simulink model "srinu_ver6"  (R2020b)
settings: Solver=ode15s  StartTime=0.0  StopTime=50  MaxStep=1.0  RelTol=1e-3
undefined symbols (not defined in the file): fn_1, jw_1, m_1, mu_1, r_1, slip_1, v_1, w
libraries: pid_lib x1
settings Model: Creator=K E S SRINIVAS  LastModifiedBy=K E S SRINIVAS

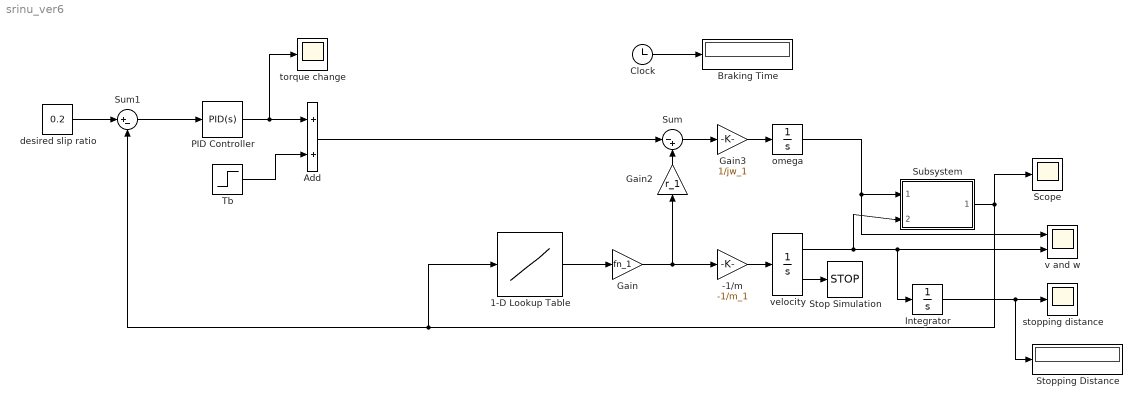
== system srinu_ver6 ==
  -1/m : Gain  Gain=-1/m_1
  1-D Lookup Table : Lookup_n-D  NumberOfTableDimensions=1  BreakpointsForDimension1=slip_1  Table=mu_1  InternalRulePriority=Speed  RndMeth=Simplest  InputSameDT=on
  Add : Sum
  Braking Time : Display
  Clock : Clock
  Gain : Gain  Gain=fn_1
  Gain2 : Gain  Gain=r_1
  Gain3 : Gain  Gain=1/jw_1
  Integrator : Integrator
  PID Controller : pid_lib/PID Controller  Controller=PID  Form=Parallel  TimeDomain=Continuous-time  UseExternalTs=off  SampleTime=-1  IntegratorMethod=Forward Euler  FilterMethod=Forward Euler  ControllerParametersSource=internal  P=250  I=10  D=5  UseFilter=on  N=100  TunerSelectOption=Transfer Function Based (PID Tuner App)  InitialConditionSource=internal  InitialConditionForIntegrator=0  InitialConditionForFilter=0  DifferentiatorICPrevScaledInput=0  ExternalReset=none  TrackingMode=off  Kt=1  LimitOutput=off  SatLimitsSource=internal  UpperSaturationLimit=inf  LowerSaturationLimit=-inf  LinearizeAsGain=on  AntiWindupMode=none  Kb=1  POutMin=[]  POutMax=[]  IOutMin=[]  IOutMax=[]  DOutMin=[]  DOutMax=[]  NOutMin=[]  NOutMax=[]  SumOutMin=[]  SumOutMax=[]  SaturationOutMin=[]  SaturationOutMax=[]  PParamMin=[]  PParamMax=[]  IParamMin=[]  IParamMax=[]  DParamMin=[]  DParamMax=[]  NParamMin=[]  NParamMax=[]  KbParamMin=[]  KbParamMax=[]  KtParamMin=[]  KtParamMax=[]  KbOutMin=[]  KbOutMax=[]  KtOutMin=[]  KtOutMax=[]  IntegratorOutMin=[]  IntegratorOutMax=[]  FilterOutMin=[]  FilterOutMax=[]  SumI1OutMin=[]  SumI1OutMax=[]  SumI2OutMin=[]  SumI2OutMax=[]  SumI3OutMin=[]  SumI3OutMax=[]  SumI4OutMin=[]  SumI4OutMax=[]  SumDOutMin=[]  SumDOutMax=[]  DifferentiatorOutMin=[]  DifferentiatorOutMax=[]  FilterDiffOutCoefMin=[]  FilterDiffOutCoefMax=[]  ReciprocalOutMin=[]  ReciprocalOutMax=[]  SumDenOutMin=[]  SumDenOutMax=[]  SumNumOutMin=[]  SumNumOutMax=[]  DivideOutMin=[]  DivideOutMax=[]  UdiffTsProdOutMin=[]  UdiffTsProdOutMax=[]  NTsProdOutMin=[]  NTsProdOutMax=[]  UintegralTsProdOutMin=[]  UintegralTsProdOutMax=[]  UngainTsProdOutMin=[]  UngainTsProdOutMax=[]  IntegratorContinuousStateAttributes=''  IntegratorStateMustResolveToSignalObject=off  IntegratorRTWStateStorageClass=Auto  FilterContinuousStateAttributes=''  FilterStateMustResolveToSignalObject=off  FilterRTWStateStorageClass=Auto  ParallelPVariant=InternalParameters  IdealPVariant=Disabled  IVariant=InternalParameters  DVariant=InternalParameters  IntegratorVariant=Continuous  SatVariant=Disabled  AWVariant=Passthrough  PCopyVariant=Disabled  TRVariant=Disabled  FdbkBlocksVariant=Forward  IdealPFdbkVariant=Disabled  SatFdbkVariant=Disabled  DerivativeFilterVariant=ContFilter  NVariant=InternalParameters  NCopyVariant=Disabled  FilterICVariant=InternalICsFilter  IntegratorICVariant=InternalICs  ExternalResetVariant=Disabled  TRSumVariant=Passthrough  SumFdbkVariant=Disabled  SumVariant=Sum_PID  TsampFilterVariant=InternalTs  TsampNgainVariant=Passthrough  TsampIntegralVariant=Passthrough  ExternalSaturationOutDataTypeStr=Inherit: Same as second input
  Scope : Scope
  Stop Simulation : Stop
  Stopping Distance : Display
  Subsystem : Subsystem
  Sum : Sum  Inputs=|-+
  Sum1 : Sum  Inputs=|+-
  Tb : Step  Time=0  After=0  SampleTime=0
  desired slip ratio : Constant  Value=0.2
  omega : Integrator  InitialCondition=w  LimitOutput=on  UpperSaturationLimit=1000  LowerSaturationLimit=0
  stopping distance : Scope
  torque change : Scope
  v and w : Scope  NumInputPorts=2
  velocity : Integrator  InitialCondition=v_1  LimitOutput=on  UpperSaturationLimit=1000  LowerSaturationLimit=0  ShowSaturationPort=on
  wires:
  Gain/1 -> Gain2/1, -1/m/1
  Gain2/1 -> Sum/2
  Add/1 -> Sum/1
  Tb/1 -> Add/2
  PID Controller/1 -> torque change/1, Add/1
  Sum/1 -> Gain3/1
  Gain3/1 -> omega/1
  -1/m/1 -> velocity/1
  velocity/1 -> Integrator/1, v and w/2, Subsystem/2(velocity)
  1-D Lookup Table/1 -> Gain/1
  velocity/2 -> Stop Simulation/1
  Subsystem/1(slip ratio) -> Scope/1, 1-D Lookup Table/1, Sum1/2
  Integrator/1 -> Stopping Distance/1, stopping distance/1
  Clock/1 -> Braking Time/1
  Sum1/1 -> PID Controller/1
  desired slip ratio/1 -> Sum1/1
  omega/1 -> v and w/1, Subsystem/1(omega)

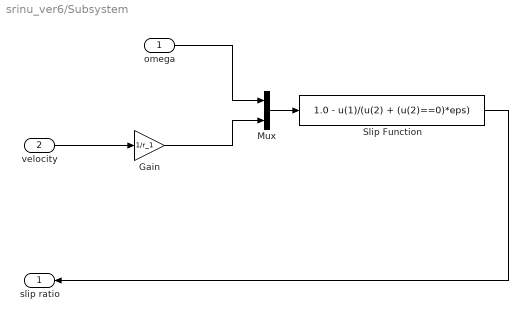
== system srinu_ver6/Subsystem ==
  omega : Inport
  velocity : Inport  Port=2
  Gain : Gain  Gain=1/r_1
  Mux : Mux  Inputs=2
  Slip Function : MATLABFcn  MATLABFcn=1.0 - u(1)/(u(2) + (u(2)==0)*eps)  OutputDimensions=1  OutputSignalType=real
  slip ratio : Outport
  wires:
  velocity/1 -> Gain/1
  Mux/1 -> Slip Function/1
  Slip Function/1 -> slip ratio/1
  omega/1 -> Mux/1
  Gain/1 -> Mux/2
